simulink model "exp6"  (Simulink 8.1)
settings: Solver=ode45  StartTime=0.0  StopTime=10.0  RelTol=1e-3
libraries: powerlib x10, simulink x6
settings Model: Creator=sidharthbatchu  LastModifiedBy=sidharthbatchu
settings DataIOCC: SignalLoggingSaveFormat=Dataset
settings OptimizationCC: ExpressionDepthLimit=128
settings DebuggingCC: FcnCallInpInsideContextMsg=EnableAllAsError
settings GRTTargetCC: CombineOutputUpdateFcns=on  GRTInterface=off

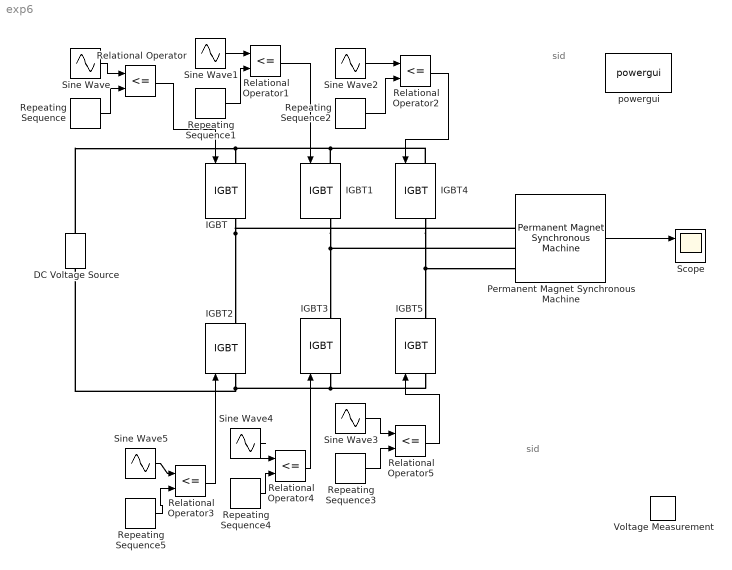
== system exp6 ==
  note: sid
  note: sid
  DC Voltage Source : powerlib/Electrical Sources/DC Voltage Source  Amplitude=100  Measurements=None
  IGBT{,1..5} (6 alike) : powerlib/Power Electronics/IGBT  Ron=0.001  Lon=0  Vf=1  Tf=1e-6  Tt=2e-6  IC=0  Rs=1e5  Cs=inf  Measurements=on
  Permanent Magnet Synchronous Machine : powerlib/Machines/Permanent Magnet Synchronous Machine  NbPhases=3  FluxDistribution=Sinusoidal  RotorType=Round  MechanicalLoad=Torque Tm  PresetModel=No  ShowDetailedParameters=on  Resistance=0.18  Inductance=8.5e-3  dqInductances=[8.5e-3,8.5e-3]  La=0.000835  MachineConstant=Flux linkage established by magnets (V.s)  Flux=0.07145  VoltageCst=51.8384  TorqueCst=0.4287  Flat=120  Mechanical=[0.00062 0.0003035 4 0]  PolePairs=4  InitialConditions=[0,0, 0,0]  InitialConditions5ph=[0 0 0 0 0 0]  TsPowergui=0  TsBlock=-1  RefAngle=90 degrees behind phase A axis (modified Park)
  Relational Operator{,1..5} (6 alike) : RelationalOperator  Operator=<=  OutDataTypeStr=boolean
  Repeating Sequence{,1..5} (6 alike) : simulink/Sources/Repeating Sequence  rep_seq_t=[0 4.76e-4 9.523e-4]  rep_seq_y=[0 1 0]
  Scope : Scope  NumInputPorts=2
      settings: YMin=-5~-5  YMax=5~5
  Sine Wave : Sin  Frequency=314.15  SampleTime=0
  Sine Wave1 : Sin  Frequency=314.159  Phase=-12.566  SampleTime=0
  Sine Wave2 : Sin  Frequency=314.159  Phase=12.566  SampleTime=0
  Sine Wave3 : Sin  Frequency=314.159  SampleTime=0
  Sine Wave4 : Sin  Frequency=314.159  SampleTime=0
  Sine Wave5 : Sin  Frequency=314.159  SampleTime=0
  Voltage Measurement : powerlib/Measurements/Voltage Measurement  PhasorSimulation=off  OutputType=Complex  PSBequivalent=0
  powergui : powerlib/powergui  Priority=1  SimulationMode=Continuous  SolverType=Tustin  SampleTime=50e-6  frequency=60  SPID=off  DisableSnubberDevices=off  DisableRonSwitches=off  DisableVfSwitches=off  SwTol=0  Interpol=off  DisplayEquations=off  frequencyindice=60  Pbase=100e6  ErrMax=1e-4  Iterations=50  UnitsV=kV  UnitsW=MW  FunctionMessages=off  echomessages=off  HookPort=off  EnableUseOfTLC=off  x0status=blocks  RestoreLinks=warning  ResistiveCurrentMeasurement=off  Frange=[0:2:500]  Ylog=off  Xlog=on  ShowGrid=off  save=off  variable=ZData  ZoomFFT=off  StartTime=0.0  cycles=1  DisplayStyle=1  fundamental=60  FreqAxis=off  MaxFrequency=1000  frequencyindicesteady=1  RmsSteady=1  display=off  Ts=0  methode=off
  wires:
  Permanent Magnet Synchronous Machine/1 -> Scope/1
  Sine Wave/1 -> Relational Operator/1
  Sine Wave5/1 -> Relational Operator3/1
  Repeating Sequence/1 -> Relational Operator/2
  Sine Wave1/1 -> Relational Operator1/1
  Repeating Sequence1/1 -> Relational Operator1/2
  Relational Operator/1 -> IGBT/1
  Relational Operator1/1 -> IGBT1/1
  Sine Wave2/1 -> Relational Operator2/1
  Repeating Sequence2/1 -> Relational Operator2/2
  Relational Operator2/1 -> IGBT4/1
  Repeating Sequence5/1 -> Relational Operator3/2
  Relational Operator3/1 -> IGBT2/1
  Sine Wave4/1 -> Relational Operator4/1
  Repeating Sequence4/1 -> Relational Operator4/2
  Relational Operator4/1 -> IGBT3/1
  Sine Wave3/1 -> Relational Operator5/1
  Repeating Sequence3/1 -> Relational Operator5/2
  Relational Operator5/1 -> IGBT5/1
  connections:
  DC Voltage Source/RConn1 -- IGBT4/LConn1 -- IGBT1/LConn1 -- IGBT/LConn1
  IGBT/RConn1 -- Permanent Magnet Synchronous Machine/LConn1 -- IGBT2/RConn1
  IGBT1/RConn1 -- IGBT3/RConn1 -- Permanent Magnet Synchronous Machine/LConn2
  IGBT2/LConn1 -- IGBT5/LConn1 -- IGBT3/LConn1 -- DC Voltage Source/LConn1
  IGBT4/RConn1 -- Permanent Magnet Synchronous Machine/LConn3 -- IGBT5/RConn1
